simulink model "ejercicio2"  (R2013a)
settings: Solver=ode45  StartTime=0.0  StopTime=10.0  RelTol=1e-3
values from neighbouring files (symbols this model uses):
  a = [0 -1;-1 0]    [Ejercicio2.m]
  b = [0;1]    [Ejercicio2.m]
  c = [1,0]    [Ejercicio2.m]
  ki = kt(1,3)    [Ejercicio2.m]
  kp = kt(1,1:2)    [Ejercicio2.m]
settings Model: Creator=mario  LastModifiedBy=mario

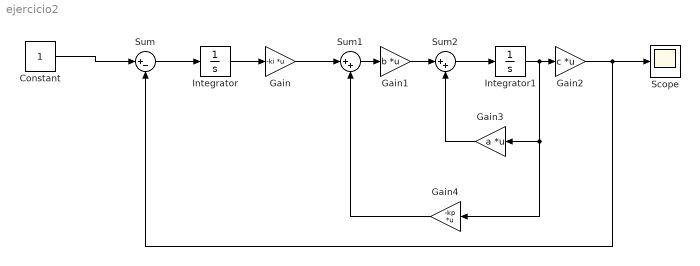
== system ejercicio2 ==
  Constant : Constant
  Gain : Gain  Gain=-ki  Multiplication=Matrix(K*u) (u vector)
  Gain1 : Gain  Gain=b  Multiplication=Matrix(K*u) (u vector)
  Gain2 : Gain  Gain=c  Multiplication=Matrix(K*u) (u vector)
  Gain3 : Gain  Gain=a  Multiplication=Matrix(K*u) (u vector)
  Gain4 : Gain  Gain=-kp  Multiplication=Matrix(K*u) (u vector)
  Integrator : Integrator
  Integrator1 : Integrator
  Scope : Scope
  Sum : Sum  Inputs=|+-
  Sum1 : Sum  Inputs=|++
  Sum2 : Sum  Inputs=|++
  wires:
  Sum/1 -> Integrator/1
  Integrator/1 -> Gain/1
  Gain/1 -> Sum1/1
  Gain4/1 -> Sum1/2
  Integrator1/1 -> Gain4/1, Gain3/1, Gain2/1
  Sum1/1 -> Gain1/1
  Gain1/1 -> Sum2/1
  Sum2/1 -> Integrator1/1
  Gain3/1 -> Sum2/2
  Gain2/1 -> Sum/2, Scope/1
  Constant/1 -> Sum/1
